simulink model "Lab5_2"  (R2022b)
settings: Solver=VariableStepAuto  StartTime=0.0  StopTime=50  RelTol=1e-3
values from neighbouring files (symbols this model uses):
  ds_des = 5    [LAB_2.m]
  J = 1.7    [LAB_2.m]
  k1e1 = 1    [LAB_2.m]
  k1e2 = 1    [LAB_2.m]
  k2e1 = 10    [LAB_2.m]
  k2e2 = 10    [LAB_2.m]
  kr = 50    [LAB_2.m]
  ks = 50    [LAB_2.m]
  kw = 20    [LAB_2.m]
  pos_init = [-10;-4;10]    [LAB_2.m]
  rot_des = axang2rotm([n_des / norm(n_des) , norm(n_des)])    [LAB_2.m]
  rot_init = axang2rotm([n_init / norm(n_init) , norm(n_init)])    [LAB_2.m]
undefined symbols (not defined in the file or in its folder): rotm2quat
libraries: matrix_library x2, uavutilslib x1
settings Model: Creator=zein  LastModifiedBy=zein

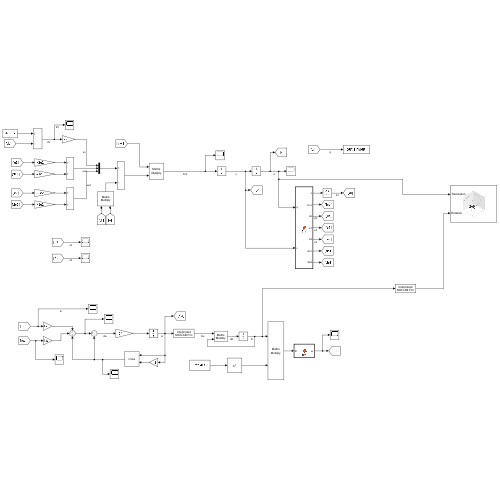
[thumbnail: Simulink's stored preview of the top-level diagram]
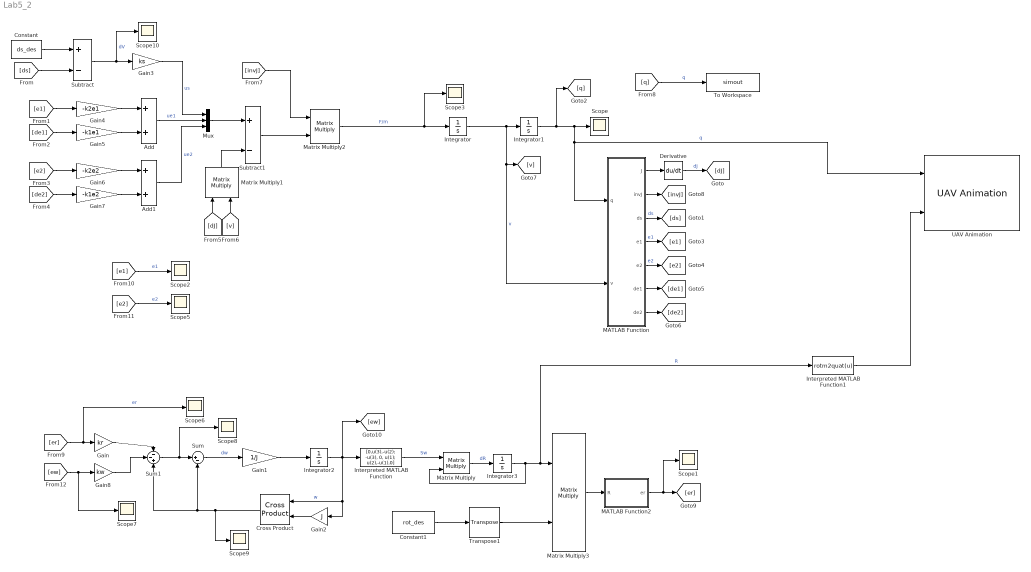
== system Lab5_2 ==
  Add : Sum
  Add1 : Sum
  Constant : Constant  Value=ds_des
  Constant1 : Constant  Value=rot_des  VectorParams1D=off
  Cross Product : matrix_library/Cross Product
  Derivative : Derivative
  Gain : Gain  Gain=kr
  Gain1 : Gain  Gain=1/J
  Gain2 : Gain  Gain=J
  Gain3 : Gain  Gain=ks
  Gain4 : Gain  Gain=-k2e1
  Gain5 : Gain  Gain=-k1e1
  Gain6 : Gain  Gain=-k2e2
  Gain7 : Gain  Gain=-k1e2
  Gain8 : Gain  Gain=kw
  Integrator : Integrator  InitialCondition=[0;0;0]
  Integrator1 : Integrator  InitialCondition=pos_init
  Integrator2 : Integrator  InitialCondition=[0;0;0]
  Integrator3 : Integrator  InitialCondition=rot_init
  Interpreted MATLAB Function : MATLABFcn  MATLABFcn=[0,u(3),-u(2); -u(3), 0, u(1); u(2),-u(1),0]  Output1D=off
  Interpreted MATLAB Function1 : MATLABFcn  MATLABFcn=rotm2quat(u)  Output1D=off
  MATLAB Function : MATLAB Function  TreatAsAtomicUnit=on
  MATLAB Function2 : MATLAB Function  TreatAsAtomicUnit=on
  Matrix Multiply{,1..3} (4 alike) : Product  Multiplication=Matrix(*)
  Mux : Mux  Inputs=3
  Scope{,1..3,5..10} (10 alike) : Scope
  Subtract : Sum  Inputs=+-
  Subtract1 : Sum  Inputs=+-
  Sum : Sum  Inputs=|+-
  Sum1 : Sum  Inputs=--+
  To Workspace : ToWorkspace  VariableName=simout  SaveFormat=Timeseries  SampleTime=-1
  Transpose1 : matrix_library/Transpose
  UAV Animation : uavutilslib/UAV Animation  UAVType=FixedWing  UAVSize=5  InertialZDirection=Up  SampleTime=-1
  wires:
  Matrix Multiply2/1 -> Scope3/1, Integrator/1  "F/m"
  Integrator/1 -> MATLAB Function/2(v), [v], Integrator1/1  "v"
  Sum1/1 -> Scope8/1, Sum/1
  Sum/1 -> Gain1/1  "dw"
  Integrator2/1 -> [ew], Gain2/1, Cross Product/1, Interpreted MATLAB Function/1  "w"
  Gain1/1 -> Integrator2/1
  Gain2/1 -> Cross Product/2
  Cross Product/1 -> Scope9/1, Sum1/3, Sum/2
  Interpreted MATLAB Function/1 -> Matrix Multiply/1  "Sw"
  Matrix Multiply/1 -> Integrator3/1  "dR"
  Integrator3/1 -> Matrix Multiply/2, Interpreted MATLAB Function1/1, Matrix Multiply3/1  "R"
  Integrator1/1 -> [q], UAV Animation/1, MATLAB Function/1(q), Scope/1  "q"
  MATLAB Function/3(ds) -> [ds]  "ds"
  MATLAB Function/1(J) -> Derivative/1
  Derivative/1 -> [dJ]  "dJ"
  MATLAB Function/4(e1) -> [e1]  "e1"
  MATLAB Function/5(e2) -> [e2]  "e2"
  Constant/1 -> Subtract/1
  [ds] -> Subtract/2
  Subtract/1 -> Scope10/1, Gain3/1  "dV"
  MATLAB Function/6(de1) -> [de1]
  MATLAB Function/7(de2) -> [de2]
  [e1] -> Gain4/1
  [de1] -> Gain5/1
  Gain4/1 -> Add/1
  Gain5/1 -> Add/2
  Gain7/1 -> Add1/2
  Gain6/1 -> Add1/1
  [de2] -> Gain7/1
  [e2] -> Gain6/1
  Gain3/1 -> Mux/1  "us"
  Add/1 -> Mux/2  "ue1"
  Add1/1 -> Mux/3  "ue2"
  Mux/1 -> Subtract1/1
  Matrix Multiply1/1 -> Subtract1/2
  [dJ] -> Matrix Multiply1/1
  [v] -> Matrix Multiply1/2
  MATLAB Function/2(invJ) -> [invJ]
  Subtract1/1 -> Matrix Multiply2/2
  [invJ] -> Matrix Multiply2/1
  Constant1/1 -> Transpose1/1
  Transpose1/1 -> Matrix Multiply3/2
  Matrix Multiply3/1 -> MATLAB Function2/1(R)
  MATLAB Function2/1(er) -> Scope1/1, [er]
  [er] -> Scope6/1, Gain/1  "er"
  Gain/1 -> Sum1/1
  [e1] -> Scope2/1  "e1"
  [e2] -> Scope5/1  "e2"
  [ew] -> Scope7/1, Gain8/1
  Gain8/1 -> Sum1/2
  Interpreted MATLAB Function1/1 -> UAV Animation/2
  [q] -> To Workspace/1  "q"

== matlab function Lab5_2/MATLAB Function ==
  data: q input; J output; invJ output; v input; ds output; e1 output; e2 output; de1 output; de2 output
function [J, invJ, ds, e1, e2, de1, de2] = fcn(q, v)

x = q(1);
y = q(2);
z = q(3);

J = [[y.*1.0./sqrt(x.^2.*2.0+y.^2);x.*1.0./sqrt(x.^2+y.^2);0.0], ...
     [-x.*1.0./sqrt(x.^2.*2.0+y.^2);y.*1.0./sqrt(x.^2+y.^2);sqrt(2.0)./2.0],...
     [x.*1.0./sqrt(x.^2.*2.0+y.^2);0.0;sqrt(2.0)./2.0]];
invJ = inv(J);

ds = J(1,:)* v;

e1 = x^2 +y^2 -400;

e2 = z+y-10;

grad_1 = [x.*2.0,y.*2.0,0.0];
grad_2 = [0.0,1.0,1.0];

de1 = grad_1 * v;
de2 = grad_2 * v;

== matlab function Lab5_2/MATLAB Function2 ==
  data: R input; er output
function er = fcn(R)

A = R - R.';

e = [A(2,3); A(3,1); A(1,2)];

er = e/2;
